simulink model "twr_2017a"  (R2020a)
settings: Solver=FixedStepDiscrete  StartTime=0.0  StopTime=inf  FixedStep=mdl_T_sample  RelTol=1e-3
undefined symbols (not defined in the file or in its folder): ctrl_lqr_addlDyn_A_discrete, ctrl_lqr_addlDyn_B_discrete, ctrl_lqr_addlDyn_C_discrete, ctrl_lqr_addlDyn_D_discrete, ctrl_lqr_addlDyn_k_antiWindup, ctrl_lqr_addlDyn_stateIC, ctrl_lqr_K2, ctrl_motorDriver_v_ff_cmd_v_val, ctrl_motorDriver_v_ff_cmd_v_val_norm_dx_max, ctrl_motorDriver_v_ff_cmd_v_val_norm_dx_min, ctrl_motorDriver_v_output_max, ctrl_motorDriver_v_output_min, ctrl_motorDriver_v_pid_cmd_thetaDot_val, ctrl_motorDriver_v_pid_cmd_thetaDot_val_norm_dx_max, ctrl_motorDriver_v_pid_cmd_thetaDot_val_norm_dx_min, ctrl_motorDriver_v_pid_int_maxVal, ctrl_motorDriver_v_pid_int_minVal, ctrl_motorDriver_v_pid_k_d, ctrl_motorDriver_v_pid_k_i, ctrl_motorDriver_v_pid_k_p, ctrl_motorDriver_v_rts_ss_k_A, ctrl_motorDriver_v_rts_ss_k_B, ctrl_motorDriver_v_rts_ss_k_C, ctrl_motorDriver_v_rts_ss_k_D, ctrl_motorDriver_v_rts_ss_stateIC, ctrl_motorDriver_v_sfr_cmd_p_x_f, ctrl_motorDriver_v_sfr_cmd_p_x_mag, ctrl_motorDriver_v_sfr_cmd_p_y_f, ctrl_motorDriver_v_sfr_cmd_p_y_mag, ctrl_motorDriver_v_sfr_K, ctrl_motorDriver_v_sfr_K_plant, ctrl_motorDriver_v_sfr_K_rts, ctrl_motorDriver_v_T_cmd, ctrl_motorDriver_v_T_init, DiscIntNeverNeededParam, gyro_bias, io_srl_read_rateTransition_initialCondition, k_intmax_uint8, mdl_T_sample, mtr_encoder_filter_z_ss_A, mtr_encoder_filter_z_ss_B, mtr_encoder_filter_z_ss_C, mtr_encoder_filter_z_ss_D, plant, plant_accel_k_digital2analog, plant_body_l_c, plant_body_l_w, plant_gyro_bias_movingAverage_n_pts, plant_gyro_encoder_filter_z_den, plant_gyro_encoder_filter_z_num, plant_gyro_filter_z_den, plant_gyro_filter_z_num, plant_gyro_k_digital2analog, plant_linear_A_continuous, plant_linear_B_continuous, plant_linear_C_continuous, plant_linear_D_continuous, plant_linear_ss_stateIC, plant_linear_ss_t_A, plant_linear_ss_t_B ... (+10)
libraries: svdutilitieslib x135, simulink x57, arduinolib x15, MinSegLibrary_M2V3 x3, dspindex x3, RASPlib x2
(part 5 of 6)

== system twr_2017a/User IO/Writes (To PC)/Plant: Linear Dynamics/Controller: PID/Motor Characterization ==
  note: There is no need to change the datatype paramter
      | listed in the Byte Pack blocks.
      |
      | It will update automatically based on the datatype parameter
      | listed in the Datatype Conversion Block,
      | through the use of the initialization script.
  systemSignalBus : Inport
  Bus Selector : BusSelector  OutputSignals="plant.clock.time [s],io.reads.userInput.controller.output_vMotor.command,plant.encoders.left.angularVelocity  [rad/s],plant.encoders.middle.angularVelocity  [rad/s],controller.motorAngularVelocity.left.voltage.command [V],controller.motorAngularVelocity.middle.voltage.command [V],plant.drivers.left.voltage.command.digital.positive [V],plant.drivers.left.voltage.command.digital.negative [V],plant.drivers.middle.voltage.command.digital.positive [V],plant.drivers.middle.voltage.command.digital.negative [V]"
  Byte Pack - 01 : svdutilitieslib/Byte Pack  datatypes={'single'}  byteAlign=1  blockPlatform=arduinoert
      settings: AttributesFormatString=%<datatypes>  SourceProductName=Simulink Support Package for Arduino Hardware
  Byte Pack - 02 : svdutilitieslib/Byte Pack  datatypes={'single'}  byteAlign=1  blockPlatform=arduinoert
      settings: AttributesFormatString=%<datatypes>  SourceProductName=Simulink Support Package for Arduino Hardware
  Byte Pack - 03 : svdutilitieslib/Byte Pack  datatypes={'single'}  byteAlign=1  blockPlatform=arduinoert
      settings: AttributesFormatString=%<datatypes>  SourceProductName=Simulink Support Package for Arduino Hardware
  Byte Pack - 04 : svdutilitieslib/Byte Pack  datatypes={'single'}  byteAlign=1  blockPlatform=arduinoert
      settings: AttributesFormatString=%<datatypes>  SourceProductName=Simulink Support Package for Arduino Hardware
  Byte Pack - 05 : svdutilitieslib/Byte Pack  datatypes={'single'}  byteAlign=1  blockPlatform=arduinoert
      settings: AttributesFormatString=%<datatypes>  SourceProductName=Simulink Support Package for Arduino Hardware
  Byte Pack - 06 : svdutilitieslib/Byte Pack  datatypes={'single'}  byteAlign=1  blockPlatform=arduinoert
      settings: AttributesFormatString=%<datatypes>  SourceProductName=Simulink Support Package for Arduino Hardware
  Byte Pack - 07 : svdutilitieslib/Byte Pack  datatypes={'single'}  byteAlign=1  blockPlatform=arduinoert
      settings: AttributesFormatString=%<datatypes>  SourceProductName=Simulink Support Package for Arduino Hardware
  Byte Pack - 08 : svdutilitieslib/Byte Pack  datatypes={'single'}  byteAlign=1  blockPlatform=arduinoert
      settings: AttributesFormatString=%<datatypes>  SourceProductName=Simulink Support Package for Arduino Hardware
  Byte Pack - 09 : svdutilitieslib/Byte Pack  datatypes={'uint8'}  byteAlign=1  blockPlatform=arduinoert
      settings: AttributesFormatString=%<datatypes>  SourceProductName=Simulink Support Package for Arduino Hardware
  Byte Pack - 10 : svdutilitieslib/Byte Pack  datatypes={'uint8'}  byteAlign=1  blockPlatform=arduinoert
      settings: AttributesFormatString=%<datatypes>  SourceProductName=Simulink Support Package for Arduino Hardware
  Data Type Conversion - 01 : DataTypeConversion  OutDataTypeStr=single
  Data Type Conversion - 02 : DataTypeConversion  OutDataTypeStr=single
  Data Type Conversion - 03 : DataTypeConversion  OutDataTypeStr=single
  Data Type Conversion - 04 : DataTypeConversion  OutDataTypeStr=single
  Data Type Conversion - 05 : DataTypeConversion  OutDataTypeStr=single
  Data Type Conversion - 06 : DataTypeConversion  OutDataTypeStr=single
  Data Type Conversion - 07 : DataTypeConversion  OutDataTypeStr=uint8
  Data Type Conversion - 08 : DataTypeConversion  OutDataTypeStr=uint8
  Data Type Conversion - 09 : DataTypeConversion  OutDataTypeStr=uint8
  Data Type Conversion - 10 : DataTypeConversion  OutDataTypeStr=uint8
  Mux : Mux  Inputs=10
  Rate Transition : RateTransition  InitialCondition=io_srl_read_rateTransition_initialCondition  OutPortSampleTimeMultiple=io_read_rateTransition_decimation  OutPortSampleTime=io_srl_read_rateTransition_T_sample
      settings: AttributesFormatString=|
      | Output sample time: %<OutPortSampleTime>
      | Initial condition: %<X0>
  Serial Transmit : arduinolib/Serial Transmit  portNumber=0  sendmode=write  sendformat=Decimal  floatprecision=2  blockPlatform=arduino
  wires:
  Bus Selector/1 -> Data Type Conversion - 01/1  "<time [s]>"
  Rate Transition/1 -> Serial Transmit/1
  Bus Selector/4 -> Data Type Conversion - 04/1  "<angularVelocity  [rad/s]>"
  Bus Selector/3 -> Data Type Conversion - 03/1  "<angularVelocity  [rad/s]>"
  Data Type Conversion - 10/1 -> Byte Pack - 10/1
  Data Type Conversion - 09/1 -> Byte Pack - 09/1
  Data Type Conversion - 08/1 -> Byte Pack - 08/1
  Data Type Conversion - 07/1 -> Byte Pack - 07/1
  Data Type Conversion - 06/1 -> Byte Pack - 06/1
  Data Type Conversion - 05/1 -> Byte Pack - 05/1
  Data Type Conversion - 04/1 -> Byte Pack - 04/1
  Data Type Conversion - 03/1 -> Byte Pack - 03/1
  Data Type Conversion - 02/1 -> Byte Pack - 02/1
  Data Type Conversion - 01/1 -> Byte Pack - 01/1
  Byte Pack - 10/1 -> Mux/10
  Byte Pack - 09/1 -> Mux/9
  Bus Selector/2 -> Data Type Conversion - 02/1  "<command>"
  systemSignalBus/1 -> Bus Selector/1
  Byte Pack - 02/1 -> Mux/2
  Byte Pack - 08/1 -> Mux/8
  Byte Pack - 05/1 -> Mux/5
  Byte Pack - 06/1 -> Mux/6
  Byte Pack - 01/1 -> Mux/1
  Mux/1 -> Rate Transition/1
  Byte Pack - 07/1 -> Mux/7
  Byte Pack - 03/1 -> Mux/3
  Byte Pack - 04/1 -> Mux/4
  Bus Selector/5 -> Data Type Conversion - 05/1  "<command [V]>"
  Bus Selector/6 -> Data Type Conversion - 06/1  "<command [V]>"
  Bus Selector/7 -> Data Type Conversion - 07/1  "<positive [V]>"
  Bus Selector/8 -> Data Type Conversion - 08/1  "<negative [V]>"
  Bus Selector/9 -> Data Type Conversion - 09/1  "<positive [V]>"
  Bus Selector/10 -> Data Type Conversion - 10/1  "<negative [V]>"

== system twr_2017a/User IO/Writes (To PC)/Plant: Linear Dynamics/Controller: PID/Standard ==
  systemSignalBus : Inport
  Bus Creator : BusCreator  Inputs=4
  Bus Selector : BusSelector  OutputSignals=userIO.read.controller.command.theta_body_average [rad],plant.position.theta.global.average.position [rad],controller.error.motorDriver.error.theta_body_average [rad]
  Bus Selector1 : BusSelector  OutputSignals=userIO.read.controller.command.phi_y [rad],plant.position.phi.y (yaw).position [rad],controller.error.motorDriver.error.phi_y [rad]
  Bus Selector2 : BusSelector  OutputSignals=plant.position.phi.x (pitch).position [rad]
  Bus Selector3 : BusSelector  OutputSignals="controller.output.motorDriver.left.voltage.command  [V],controller.output.motorDriver.middle.voltage.command [V]"
  Bus Selector4 : BusSelector  OutputSignals=plant.position.p.wheel.center.x.position [m],plant.position.p.wheel.center.y.position [m]
  Bus Selector5 : BusSelector  OutputSignals=plant.position.p.wheel.center.x.position [m],plant.position.p.wheel.center.y.position [m]
  Bus Selector6 : BusSelector  OutputSignals=userIO.read.controller.command.theta_body_average [rad],userIO.read.controller.command.phi_y [rad]
  Bus Selector7 : BusSelector  OutputSignals=x.position [m],y.position [m]
  Bus Selector8 : BusSelector  OutputSignals=plant.position.p.wheel.center.x.position [m],plant.position.p.wheel.center.y.position [m]
  Discrete Derivative : simulink/Discrete/Discrete Derivative  gainval=1.0  ICPrevScaledInput=0.0  OutMin=[]  OutMax=[]  OutDataType=fixdt(1, 16)  OutScaling=2^-10  DoSatur=off
  Pass Through : Subsystem
  To Workspace : ToWorkspace  VariableName=xy  SaveFormat=Timeseries  SampleTime=-1
  Wheel : Subsystem
  XY Graph : simulink/Sinks/XY Graph  xmin=-1  xmax=+1  ymin=-1  ymax=+1  st=-1
  pitch : Scope
  theta : Scope  NumInputPorts=3
  v.lm : Scope  NumInputPorts=2
  xy : Scope  NumInputPorts=2
  yaw : Scope  NumInputPorts=3
  wires:
  Bus Selector/1 -> theta/1  "<theta_body_average [rad]>"
  Bus Selector/2 -> theta/2  "<position [rad]>"
  Bus Selector/3 -> theta/3  "<theta_body_average [rad]>"
  Bus Selector1/1 -> yaw/1  "<phi_y [rad]>"
  Bus Selector1/2 -> yaw/2  "<position [rad]>"
  Bus Selector1/3 -> yaw/3  "<phi_y [rad]>"
  Bus Selector2/1 -> pitch/1  "<position [rad]>"
  Bus Selector3/1 -> v.lm/1  "<command  [V]>"
  Bus Selector3/2 -> v.lm/2  "<command [V]>"
  Bus Selector5/1 -> xy/1  "<position [m]>"
  Bus Selector5/2 -> xy/2  "<position [m]>"
  Bus Selector4/2 -> XY Graph/2  "<position [m]>"
  Bus Selector4/1 -> XY Graph/1  "<position [m]>"
  Bus Selector6/1 -> Discrete Derivative/1  "<theta_body_average [rad]>"
  Bus Selector6/2 -> Wheel/2(body.angularPosition.y (yaw))  "<phi_y [rad]>"
  Wheel/3(center) -> Bus Selector7/1
  Discrete Derivative/1 -> Wheel/1(wheel.angularVelocity.global)
  systemSignalBus/1 -> Bus Selector5/1, Bus Selector4/1, Bus Selector6/1, Bus Selector8/1, Bus Selector3/1, Bus Selector2/1, Bus Selector1/1, Bus Selector/1
  Pass Through/4(Out4) -> Bus Creator/4  "act.y"
  Pass Through/3(Out3) -> Bus Creator/3  "act.x"
  Pass Through/2(Out2) -> Bus Creator/2  "ref.y"
  Pass Through/1(Out1) -> Bus Creator/1  "ref.x"
  Bus Creator/1 -> To Workspace/1
  Bus Selector7/1 -> Pass Through/1(In1)  "<position [m]>"
  Bus Selector7/2 -> Pass Through/2(In2)  "<position [m]>"
  Bus Selector8/1 -> Pass Through/3(In3)  "<position [m]>"
  Bus Selector8/2 -> Pass Through/4(In4)  "<position [m]>"

== system twr_2017a/User IO/Writes (To PC)/Plant: Linear Dynamics/Controller: SFR/Error ==
  x.command.in : Inport
  y.command.in : Inport  Port=2
  x.actual.in : Inport  Port=3
  y.actual.in : Inport  Port=4
  Add : Sum  Inputs=+-
  Add1 : Sum  Inputs=+-
  x.command : Outport
  x.actual : Outport  Port=2
  x.error : Outport  Port=3
  y.command : Outport  Port=4
  y.actual : Outport  Port=5
  y.error : Outport  Port=6
  wires:
  x.command.in/1 -> [x_cmd]
  x.actual.in/1 -> [x_act]
  y.command.in/1 -> [y_cmd]
  y.actual.in/1 -> [y_act]
  [x_cmd] -> x.command/1
  [x_act] -> x.actual/1
  [y_cmd] -> y.command/1
  [y_act] -> y.actual/1
  Add/1 -> y.error/1
  [y_cmd] -> Add/1
  [y_act] -> Add/2
  [x_act] -> Add1/2
  [x_cmd] -> Add1/1
  Add1/1 -> x.error/1

== system twr_2017a/User IO/Writes (To PC)/Plant: Nonlinear Dynamics/Controller: FF/Standard ==
  note: There is no need to change the datatype paramter
      | listed in the Byte Pack blocks.
      |
      | It will update automatically based on the datatype parameter
      | listed in the Datatype Conversion Block,
      | through the use of the initialization script.
  systemSignalBus : Inport
  Bus Selector : BusSelector  OutputSignals="plant.clock.time [s],io.reads.userInput.command,plant.encoders.left.angularVelocity  [rad/s],plant.encoders.middle.angularVelocity  [rad/s],controller.motorAngularVelocity.left.voltage.command [V],controller.motorAngularVelocity.middle.voltage.command [V],plant.drivers.left.voltage.command.digital.positive [V],plant.drivers.left.voltage.command.digital.negative [V],plant.drivers.middle.voltage.command.digital.positive [V],plant.drivers.middle.voltage.command.digital.negative [V],plant.gyroscope.x.w [rad/s],plant.gyroscope.x.theta [rad],plant.gyroscope.y.w [rad/s],plant.gyroscope.y.theta [rad],plant.gyroscope.z.w [rad/s],plant.gyroscope.z.theta [rad]"
  Byte Pack - 01 : svdutilitieslib/Byte Pack  datatypes={'single'}  byteAlign=1  blockPlatform=arduinoert
      settings: AttributesFormatString=%<datatypes>  SourceProductName=Simulink Support Package for Arduino Hardware
  Byte Pack - 02 : svdutilitieslib/Byte Pack  datatypes={'single'}  byteAlign=1  blockPlatform=arduinoert
      settings: AttributesFormatString=%<datatypes>  SourceProductName=Simulink Support Package for Arduino Hardware
  Byte Pack - 03 : svdutilitieslib/Byte Pack  datatypes={'single'}  byteAlign=1  blockPlatform=arduinoert
      settings: AttributesFormatString=%<datatypes>  SourceProductName=Simulink Support Package for Arduino Hardware
  Byte Pack - 04 : svdutilitieslib/Byte Pack  datatypes={'single'}  byteAlign=1  blockPlatform=arduinoert
      settings: AttributesFormatString=%<datatypes>  SourceProductName=Simulink Support Package for Arduino Hardware
  Byte Pack - 05 : svdutilitieslib/Byte Pack  datatypes={'single'}  byteAlign=1  blockPlatform=arduinoert
      settings: AttributesFormatString=%<datatypes>  SourceProductName=Simulink Support Package for Arduino Hardware
  Byte Pack - 06 : svdutilitieslib/Byte Pack  datatypes={'single'}  byteAlign=1  blockPlatform=arduinoert
      settings: AttributesFormatString=%<datatypes>  SourceProductName=Simulink Support Package for Arduino Hardware
  Byte Pack - 07 : svdutilitieslib/Byte Pack  datatypes={'single'}  byteAlign=1  blockPlatform=arduinoert
      settings: AttributesFormatString=%<datatypes>  SourceProductName=Simulink Support Package for Arduino Hardware
  Byte Pack - 08 : svdutilitieslib/Byte Pack  datatypes={'single'}  byteAlign=1  blockPlatform=arduinoert
      settings: AttributesFormatString=%<datatypes>  SourceProductName=Simulink Support Package for Arduino Hardware
  Byte Pack - 09 : svdutilitieslib/Byte Pack  datatypes={'uint8'}  byteAlign=1  blockPlatform=arduinoert
      settings: AttributesFormatString=%<datatypes>  SourceProductName=Simulink Support Package for Arduino Hardware
  Byte Pack - 10 : svdutilitieslib/Byte Pack  datatypes={'uint8'}  byteAlign=1  blockPlatform=arduinoert
      settings: AttributesFormatString=%<datatypes>  SourceProductName=Simulink Support Package for Arduino Hardware
  Byte Pack - 11 : svdutilitieslib/Byte Pack  datatypes={'uint8'}  byteAlign=1  blockPlatform=arduinoert
      settings: AttributesFormatString=%<datatypes>  SourceProductName=Simulink Support Package for Arduino Hardware
  Byte Pack - 12 : svdutilitieslib/Byte Pack  datatypes={'uint8'}  byteAlign=1  blockPlatform=arduinoert
      settings: AttributesFormatString=%<datatypes>  SourceProductName=Simulink Support Package for Arduino Hardware
  Byte Pack - 13 : svdutilitieslib/Byte Pack  datatypes={'single'}  byteAlign=1  blockPlatform=arduinoert
      settings: AttributesFormatString=%<datatypes>  SourceProductName=Simulink Support Package for Arduino Hardware
  Byte Pack - 14 : svdutilitieslib/Byte Pack  datatypes={'single'}  byteAlign=1  blockPlatform=arduinoert
      settings: AttributesFormatString=%<datatypes>  SourceProductName=Simulink Support Package for Arduino Hardware
  Data Type Conversion - 01 : DataTypeConversion  OutDataTypeStr=single
  Data Type Conversion - 02 : DataTypeConversion  OutDataTypeStr=single
  Data Type Conversion - 03 : DataTypeConversion  OutDataTypeStr=single
  Data Type Conversion - 04 : DataTypeConversion  OutDataTypeStr=single
  Data Type Conversion - 05 : DataTypeConversion  OutDataTypeStr=single
  Data Type Conversion - 06 : DataTypeConversion  OutDataTypeStr=single
  Data Type Conversion - 07 : DataTypeConversion  OutDataTypeStr=single
  Data Type Conversion - 08 : DataTypeConversion  OutDataTypeStr=single
  Data Type Conversion - 09 : DataTypeConversion  OutDataTypeStr=uint8
  Data Type Conversion - 10 : DataTypeConversion  OutDataTypeStr=uint8
  Data Type Conversion - 11 : DataTypeConversion  OutDataTypeStr=uint8
  Data Type Conversion - 12 : DataTypeConversion  OutDataTypeStr=uint8
  Data Type Conversion - 13 : DataTypeConversion  OutDataTypeStr=single
  Data Type Conversion - 14 : DataTypeConversion  OutDataTypeStr=single
  Mux : Mux  Inputs=14
  Rate Transition : RateTransition  InitialCondition=io_srl_read_rateTransition_initialCondition  OutPortSampleTimeMultiple=io_read_rateTransition_decimation  OutPortSampleTime=io_srl_read_rateTransition_T_sample
      settings: AttributesFormatString=|
      | Output sample time: %<OutPortSampleTime>
      | Initial condition: %<X0>
  Serial Transmit : arduinolib/Serial Transmit  portNumber=0  sendmode=write  sendformat=Decimal  floatprecision=2  blockPlatform=arduino
  wires:
  Bus Selector/1 -> Data Type Conversion - 01/1  "<time [s]>"
  Byte Pack - 14/1 -> Mux/14
  Bus Selector/12 -> Data Type Conversion - 14/1  "<theta [rad]>"
  Data Type Conversion - 14/1 -> Byte Pack - 14/1
  Bus Selector/11 -> Data Type Conversion - 13/1  "<w [rad/s]>"
  Data Type Conversion - 13/1 -> Byte Pack - 13/1
  Byte Pack - 13/1 -> Mux/13
  Rate Transition/1 -> Serial Transmit/1
  Bus Selector/6 -> Data Type Conversion - 08/1  "<command [V]>"
  Bus Selector/5 -> Data Type Conversion - 07/1  "<command [V]>"
  ? -> Data Type Conversion - 06/1  "<error [rad/s]>"
  ? -> Data Type Conversion - 05/1  "<error [rad/s]>"
  Bus Selector/4 -> Data Type Conversion - 04/1  "<angularVelocity  [rad/s]>"
  Bus Selector/3 -> Data Type Conversion - 03/1  "<angularVelocity  [rad/s]>"
  Byte Pack - 12/1 -> Mux/12
  Byte Pack - 11/1 -> Mux/11
  Bus Selector/9 -> Data Type Conversion - 11/1  "<positive [V]>"
  Bus Selector/10 -> Data Type Conversion - 12/1  "<negative [V]>"
  Data Type Conversion - 11/1 -> Byte Pack - 11/1
  Data Type Conversion - 12/1 -> Byte Pack - 12/1
  Data Type Conversion - 10/1 -> Byte Pack - 10/1
  Data Type Conversion - 09/1 -> Byte Pack - 09/1
  Data Type Conversion - 08/1 -> Byte Pack - 08/1
  Data Type Conversion - 07/1 -> Byte Pack - 07/1
  Data Type Conversion - 06/1 -> Byte Pack - 06/1
  Data Type Conversion - 05/1 -> Byte Pack - 05/1
  Data Type Conversion - 04/1 -> Byte Pack - 04/1
  Data Type Conversion - 03/1 -> Byte Pack - 03/1
  Data Type Conversion - 02/1 -> Byte Pack - 02/1
  Data Type Conversion - 01/1 -> Byte Pack - 01/1
  Byte Pack - 10/1 -> Mux/10
  Byte Pack - 09/1 -> Mux/9
  Bus Selector/8 -> Data Type Conversion - 10/1  "<negative [V]>"
  Bus Selector/7 -> Data Type Conversion - 09/1  "<positive [V]>"
  Bus Selector/2 -> Data Type Conversion - 02/1  "<command>"
  systemSignalBus/1 -> Bus Selector/1
  Byte Pack - 02/1 -> Mux/2
  Byte Pack - 08/1 -> Mux/8
  Byte Pack - 05/1 -> Mux/5
  Byte Pack - 06/1 -> Mux/6
  Byte Pack - 01/1 -> Mux/1
  Mux/1 -> Rate Transition/1
  Byte Pack - 07/1 -> Mux/7
  Byte Pack - 03/1 -> Mux/3
  Byte Pack - 04/1 -> Mux/4

== system twr_2017a/User IO/Writes (To PC)/Plant: Nonlinear Dynamics/Controller: PID/Standard ==
  note: There is no need to change the datatype paramter
      | listed in the Byte Pack blocks.
      |
      | It will update automatically based on the datatype parameter
      | listed in the Datatype Conversion Block,
      | through the use of the initialization script.
  systemSignalBus : Inport
  Bus Selector : BusSelector  OutputSignals="plant.clock.time [s],io.reads.userInput.command,plant.encoders.left.angularVelocity  [rad/s],plant.encoders.middle.angularVelocity  [rad/s],controller.motorAngularVelocity.left.voltage.command [V],controller.motorAngularVelocity.middle.voltage.command [V],plant.drivers.left.voltage.command.digital.positive [V],plant.drivers.left.voltage.command.digital.negative [V],plant.drivers.middle.voltage.command.digital.positive [V],plant.drivers.middle.voltage.command.digital.negative [V],plant.gyroscope.x.w [rad/s],plant.gyroscope.x.theta [rad],plant.gyroscope.y.w [rad/s],plant.gyroscope.y.theta [rad],plant.gyroscope.z.w [rad/s],plant.gyroscope.z.theta [rad]"
  Byte Pack - 01 : svdutilitieslib/Byte Pack  datatypes={'single'}  byteAlign=1  blockPlatform=arduinoert
      settings: AttributesFormatString=%<datatypes>  SourceProductName=Simulink Support Package for Arduino Hardware
  Byte Pack - 02 : svdutilitieslib/Byte Pack  datatypes={'single'}  byteAlign=1  blockPlatform=arduinoert
      settings: AttributesFormatString=%<datatypes>  SourceProductName=Simulink Support Package for Arduino Hardware
  Byte Pack - 03 : svdutilitieslib/Byte Pack  datatypes={'single'}  byteAlign=1  blockPlatform=arduinoert
      settings: AttributesFormatString=%<datatypes>  SourceProductName=Simulink Support Package for Arduino Hardware
  Byte Pack - 04 : svdutilitieslib/Byte Pack  datatypes={'single'}  byteAlign=1  blockPlatform=arduinoert
      settings: AttributesFormatString=%<datatypes>  SourceProductName=Simulink Support Package for Arduino Hardware
  Byte Pack - 05 : svdutilitieslib/Byte Pack  datatypes={'single'}  byteAlign=1  blockPlatform=arduinoert
      settings: AttributesFormatString=%<datatypes>  SourceProductName=Simulink Support Package for Arduino Hardware
  Byte Pack - 06 : svdutilitieslib/Byte Pack  datatypes={'single'}  byteAlign=1  blockPlatform=arduinoert
      settings: AttributesFormatString=%<datatypes>  SourceProductName=Simulink Support Package for Arduino Hardware
  Byte Pack - 07 : svdutilitieslib/Byte Pack  datatypes={'single'}  byteAlign=1  blockPlatform=arduinoert
      settings: AttributesFormatString=%<datatypes>  SourceProductName=Simulink Support Package for Arduino Hardware
  Byte Pack - 08 : svdutilitieslib/Byte Pack  datatypes={'single'}  byteAlign=1  blockPlatform=arduinoert
      settings: AttributesFormatString=%<datatypes>  SourceProductName=Simulink Support Package for Arduino Hardware
  Byte Pack - 09 : svdutilitieslib/Byte Pack  datatypes={'uint8'}  byteAlign=1  blockPlatform=arduinoert
      settings: AttributesFormatString=%<datatypes>  SourceProductName=Simulink Support Package for Arduino Hardware
  Byte Pack - 10 : svdutilitieslib/Byte Pack  datatypes={'uint8'}  byteAlign=1  blockPlatform=arduinoert
      settings: AttributesFormatString=%<datatypes>  SourceProductName=Simulink Support Package for Arduino Hardware
  Byte Pack - 11 : svdutilitieslib/Byte Pack  datatypes={'uint8'}  byteAlign=1  blockPlatform=arduinoert
      settings: AttributesFormatString=%<datatypes>  SourceProductName=Simulink Support Package for Arduino Hardware
  Byte Pack - 12 : svdutilitieslib/Byte Pack  datatypes={'uint8'}  byteAlign=1  blockPlatform=arduinoert
      settings: AttributesFormatString=%<datatypes>  SourceProductName=Simulink Support Package for Arduino Hardware
  Byte Pack - 13 : svdutilitieslib/Byte Pack  datatypes={'single'}  byteAlign=1  blockPlatform=arduinoert
      settings: AttributesFormatString=%<datatypes>  SourceProductName=Simulink Support Package for Arduino Hardware
  Byte Pack - 14 : svdutilitieslib/Byte Pack  datatypes={'single'}  byteAlign=1  blockPlatform=arduinoert
      settings: AttributesFormatString=%<datatypes>  SourceProductName=Simulink Support Package for Arduino Hardware
  Data Type Conversion - 01 : DataTypeConversion  OutDataTypeStr=single
  Data Type Conversion - 02 : DataTypeConversion  OutDataTypeStr=single
  Data Type Conversion - 03 : DataTypeConversion  OutDataTypeStr=single
  Data Type Conversion - 04 : DataTypeConversion  OutDataTypeStr=single
  Data Type Conversion - 05 : DataTypeConversion  OutDataTypeStr=single
  Data Type Conversion - 06 : DataTypeConversion  OutDataTypeStr=single
  Data Type Conversion - 07 : DataTypeConversion  OutDataTypeStr=single
  Data Type Conversion - 08 : DataTypeConversion  OutDataTypeStr=single
  Data Type Conversion - 09 : DataTypeConversion  OutDataTypeStr=uint8
  Data Type Conversion - 10 : DataTypeConversion  OutDataTypeStr=uint8
  Data Type Conversion - 11 : DataTypeConversion  OutDataTypeStr=uint8
  Data Type Conversion - 12 : DataTypeConversion  OutDataTypeStr=uint8
  Data Type Conversion - 13 : DataTypeConversion  OutDataTypeStr=single
  Data Type Conversion - 14 : DataTypeConversion  OutDataTypeStr=single
  Mux : Mux  Inputs=14
  Rate Transition : RateTransition  InitialCondition=io_srl_read_rateTransition_initialCondition  OutPortSampleTimeMultiple=io_read_rateTransition_decimation  OutPortSampleTime=io_srl_read_rateTransition_T_sample
      settings: AttributesFormatString=|
      | Output sample time: %<OutPortSampleTime>
      | Initial condition: %<X0>
  Serial Transmit : arduinolib/Serial Transmit  portNumber=0  sendmode=write  sendformat=Decimal  floatprecision=2  blockPlatform=arduino
  wires:
  Byte Pack - 04/1 -> Mux/4
  Byte Pack - 03/1 -> Mux/3
  Byte Pack - 07/1 -> Mux/7
  Mux/1 -> Rate Transition/1
  Byte Pack - 01/1 -> Mux/1
  Byte Pack - 06/1 -> Mux/6
  Byte Pack - 05/1 -> Mux/5
  Byte Pack - 08/1 -> Mux/8
  Byte Pack - 02/1 -> Mux/2
  systemSignalBus/1 -> Bus Selector/1
  Bus Selector/2 -> Data Type Conversion - 02/1  "<command>"
  Bus Selector/7 -> Data Type Conversion - 09/1  "<positive [V]>"
  Bus Selector/8 -> Data Type Conversion - 10/1  "<negative [V]>"
  Byte Pack - 09/1 -> Mux/9
  Byte Pack - 10/1 -> Mux/10
  Data Type Conversion - 01/1 -> Byte Pack - 01/1
  Data Type Conversion - 02/1 -> Byte Pack - 02/1
  Data Type Conversion - 03/1 -> Byte Pack - 03/1
  Data Type Conversion - 04/1 -> Byte Pack - 04/1
  Data Type Conversion - 05/1 -> Byte Pack - 05/1
  Data Type Conversion - 06/1 -> Byte Pack - 06/1
  Data Type Conversion - 07/1 -> Byte Pack - 07/1
  Data Type Conversion - 08/1 -> Byte Pack - 08/1
  Data Type Conversion - 09/1 -> Byte Pack - 09/1
  Data Type Conversion - 10/1 -> Byte Pack - 10/1
  Data Type Conversion - 12/1 -> Byte Pack - 12/1
  Data Type Conversion - 11/1 -> Byte Pack - 11/1
  Bus Selector/10 -> Data Type Conversion - 12/1  "<negative [V]>"
  Bus Selector/9 -> Data Type Conversion - 11/1  "<positive [V]>"
  Byte Pack - 11/1 -> Mux/11
  Byte Pack - 12/1 -> Mux/12
  Bus Selector/3 -> Data Type Conversion - 03/1  "<angularVelocity  [rad/s]>"
  Bus Selector/4 -> Data Type Conversion - 04/1  "<angularVelocity  [rad/s]>"
  ? -> Data Type Conversion - 05/1  "<error [rad/s]>"
  ? -> Data Type Conversion - 06/1  "<error [rad/s]>"
  Bus Selector/5 -> Data Type Conversion - 07/1  "<command [V]>"
  Bus Selector/6 -> Data Type Conversion - 08/1  "<command [V]>"
  Rate Transition/1 -> Serial Transmit/1
  Byte Pack - 13/1 -> Mux/13
  Data Type Conversion - 13/1 -> Byte Pack - 13/1
  Bus Selector/11 -> Data Type Conversion - 13/1  "<w [rad/s]>"
  Data Type Conversion - 14/1 -> Byte Pack - 14/1
  Bus Selector/12 -> Data Type Conversion - 14/1  "<theta [rad]>"
  Byte Pack - 14/1 -> Mux/14
  Bus Selector/1 -> Data Type Conversion - 01/1  "<time [s]>"

== system twr_2017a/Controller [v.motorDriver]/Archive/Additional Dynamics: Reference Tracking/Delay/x1/Saturation flag ==
  u[k+1] : Inport
  u.max : Inport  Port=2
  u.min : Inport  Port=3
  Add : Sum
  Data Type Conversion : DataTypeConversion  OutDataTypeStr=uint8
  Data Type Conversion1 : DataTypeConversion  OutDataTypeStr=uint8
  Gain : Gain  Gain=uint8(1)  OutDataTypeStr=uint8
      settings: AttributesFormatString=%<Gain>
  Gain1 : Gain  Gain=uint8(2)  OutDataTypeStr=uint8
      settings: AttributesFormatString=%<Gain>
  Relational Operator : RelationalOperator  OutDataTypeStr=boolean  RndMeth=Nearest
  Relational Operator1 : RelationalOperator  Operator=<=  OutDataTypeStr=boolean  RndMeth=Nearest
  x.saturating : Outport
  wires:
  u[k+1]/1 -> [u_kp1]
  [u_kp1] -> Relational Operator/1
  u.max/1 -> Relational Operator/2
  [u_kp1] -> Relational Operator1/1
  u.min/1 -> Relational Operator1/2
  Add/1 -> x.saturating/1  "x.saturating"
  Relational Operator1/1 -> Data Type Conversion1/1  "x.lowerSaturating"
  Relational Operator/1 -> Data Type Conversion/1  "x.upperSaturating"
  Data Type Conversion/1 -> Gain/1
  Data Type Conversion1/1 -> Gain1/1
  Gain/1 -> Add/1
  Gain1/1 -> Add/2

== system twr_2017a/Controller [v.motorDriver]/Archive/Additional Dynamics: Reference Tracking/Delay/x1/anti-windup ==
  u[k+1].preSat.in : Inport
  u[k+1].postSat.in : Inport  Port=2
  Add : Sum  Inputs=-+
  Add1 : Sum
  Gain : Gain  Gain=k_antiWindup
      settings: AttributesFormatString=%<Gain>
  u[k+1].postSat.out : Outport
  wires:
  Add1/1 -> u[k+1].postSat.out/1
  Add/1 -> Gain/1
  u[k+1].preSat.in/1 -> Add/1, Add1/1
  u[k+1].postSat.in/1 -> Add/2
  Gain/1 -> Add1/2

== system twr_2017a/Controller [v.motorDriver]/Archive/Additional Dynamics: Reference Tracking/Delay/x2/Saturation flag ==
  u[k+1] : Inport
  u.max : Inport  Port=2
  u.min : Inport  Port=3
  Add : Sum
  Data Type Conversion : DataTypeConversion  OutDataTypeStr=uint8
  Data Type Conversion1 : DataTypeConversion  OutDataTypeStr=uint8
  Gain : Gain  Gain=uint8(1)  OutDataTypeStr=uint8
      settings: AttributesFormatString=%<Gain>
  Gain1 : Gain  Gain=uint8(2)  OutDataTypeStr=uint8
      settings: AttributesFormatString=%<Gain>
  Relational Operator : RelationalOperator  OutDataTypeStr=boolean  RndMeth=Nearest
  Relational Operator1 : RelationalOperator  Operator=<=  OutDataTypeStr=boolean  RndMeth=Nearest
  x.saturating : Outport
  wires:
  Gain1/1 -> Add/2
  Gain/1 -> Add/1
  Data Type Conversion1/1 -> Gain1/1
  Data Type Conversion/1 -> Gain/1
  Relational Operator/1 -> Data Type Conversion/1  "x.upperSaturating"
  Relational Operator1/1 -> Data Type Conversion1/1  "x.lowerSaturating"
  Add/1 -> x.saturating/1  "x.saturating"
  u.min/1 -> Relational Operator1/2
  [u_kp1] -> Relational Operator1/1
  u.max/1 -> Relational Operator/2
  [u_kp1] -> Relational Operator/1
  u[k+1]/1 -> [u_kp1]

== system twr_2017a/Controller [v.motorDriver]/Archive/Additional Dynamics: Reference Tracking/Delay/x2/anti-windup ==
  u[k+1].preSat.in : Inport
  u[k+1].postSat.in : Inport  Port=2
  Add : Sum  Inputs=-+
  Add1 : Sum
  Gain : Gain  Gain=k_antiWindup
      settings: AttributesFormatString=%<Gain>
  u[k+1].postSat.out : Outport
  wires:
  Gain/1 -> Add1/2
  u[k+1].postSat.in/1 -> Add/2
  u[k+1].preSat.in/1 -> Add1/1, Add/1
  Add/1 -> Gain/1
  Add1/1 -> u[k+1].postSat.out/1

== system twr_2017a/Controller [v.motorDriver]/Archive/Continuous State-Space/Integrator/x1/Saturation flag ==
  u.dot : Inport
  u.max : Inport  Port=2
  u.noSat : Inport  Port=3
  u.min : Inport  Port=4
  Compare To Zero : simulink/Logic and Bit Operations/Compare To Zero  relop=<  OutDataTypeStr=uint8  ZeroCross=off
  Compare To Zero1 : simulink/Logic and Bit Operations/Compare To Zero  relop=>  OutDataTypeStr=uint8  ZeroCross=off
  Logical Operator : Logic  Operator=OR  AllPortsSameDT=off  OutDataTypeStr=boolean
  Logical Operator1 : Logic  Operator=OR  AllPortsSameDT=off  OutDataTypeStr=boolean
  Logical Operator2 : Logic  AllPortsSameDT=off  OutDataTypeStr=boolean
  Logical Operator3 : Logic  Operator=NOT  AllPortsSameDT=off  OutDataTypeStr=boolean
  Relational Operator : RelationalOperator  Operator=<=  OutDataTypeStr=boolean  RndMeth=Nearest
  Relational Operator1 : RelationalOperator  OutDataTypeStr=boolean  RndMeth=Nearest
  x.saturating : Outport
  wires:
  Logical Operator3/1 -> x.saturating/1  "x.saturating"
  [u_min] -> Relational Operator1/2
  [u_noSat] -> Relational Operator1/1
  [u_max] -> Relational Operator/2
  [u_noSat] -> Relational Operator/1
  [u_dot] -> Compare To Zero/1
  [u_dot] -> Compare To Zero1/1
  u.noSat/1 -> [u_noSat]
  Logical Operator2/1 -> Logical Operator3/1  "x.notSaturating"
  Logical Operator/1 -> Logical Operator2/1
  Logical Operator1/1 -> Logical Operator2/2
  Relational Operator1/1 -> Logical Operator1/1
  Compare To Zero1/1 -> Logical Operator1/2
  Compare To Zero/1 -> Logical Operator/2
  Relational Operator/1 -> Logical Operator/1
  u.max/1 -> [u_max]
  u.dot/1 -> [u_dot]
  u.min/1 -> [u_min]

== system twr_2017a/Controller [v.motorDriver]/Archive/Continuous State-Space/Integrator/x2/Saturation flag ==
  u.dot : Inport
  u.max : Inport  Port=2
  u.noSat : Inport  Port=3
  u.min : Inport  Port=4
  Compare To Zero : simulink/Logic and Bit Operations/Compare To Zero  relop=<  OutDataTypeStr=uint8  ZeroCross=off
  Compare To Zero1 : simulink/Logic and Bit Operations/Compare To Zero  relop=>  OutDataTypeStr=uint8  ZeroCross=off
  Logical Operator : Logic  Operator=OR  AllPortsSameDT=off  OutDataTypeStr=boolean
  Logical Operator1 : Logic  Operator=OR  AllPortsSameDT=off  OutDataTypeStr=boolean
  Logical Operator2 : Logic  AllPortsSameDT=off  OutDataTypeStr=boolean
  Logical Operator3 : Logic  Operator=NOT  AllPortsSameDT=off  OutDataTypeStr=boolean
  Relational Operator : RelationalOperator  Operator=<=  OutDataTypeStr=boolean  RndMeth=Nearest
  Relational Operator1 : RelationalOperator  OutDataTypeStr=boolean  RndMeth=Nearest
  x.saturating : Outport
  wires:
  u.min/1 -> [u_min]
  u.dot/1 -> [u_dot]
  u.max/1 -> [u_max]
  Relational Operator/1 -> Logical Operator/1
  Compare To Zero/1 -> Logical Operator/2
  Compare To Zero1/1 -> Logical Operator1/2
  Relational Operator1/1 -> Logical Operator1/1
  Logical Operator1/1 -> Logical Operator2/2
  Logical Operator/1 -> Logical Operator2/1
  Logical Operator2/1 -> Logical Operator3/1  "x.notSaturating"
  u.noSat/1 -> [u_noSat]
  [u_dot] -> Compare To Zero1/1
  [u_dot] -> Compare To Zero/1
  [u_noSat] -> Relational Operator/1
  [u_max] -> Relational Operator/2
  [u_noSat] -> Relational Operator1/1
  [u_min] -> Relational Operator1/2
  Logical Operator3/1 -> x.saturating/1  "x.saturating"

== system twr_2017a/Plant/Hardware/Arduino Pin IO/Digital Outputs (Writes to Pins)/Motor/Left-Connected ==
  motor.left.voltage.command.digital.positive : Inport
  motor.left.voltage.command.digital.negative : Inport  Port=2
  Digital Output (PWM): Pin 6 Motor Driver - Voltage Command (Positive) : arduinolib/PWM  pinNumber=6  blockPlatform=arduino
  Digital Output (PWM): Pin 8 Motor Driver - Voltage Command (Negative) : arduinolib/PWM  pinNumber=8  blockPlatform=arduino
  wires:
  motor.left.voltage.command.digital.negative/1 -> Digital Output (PWM): Pin 8 Motor Driver - Voltage Command (Negative)/1
  motor.left.voltage.command.digital.positive/1 -> Digital Output (PWM): Pin 6 Motor Driver - Voltage Command (Positive)/1

== system twr_2017a/Plant/Hardware/Arduino Pin IO/Digital Outputs (Writes to Pins)/Motor/Right-Connected ==
  motor.middle.voltage.command.digital.positive : Inport
  motor.middle.voltage.command.digital.negative : Inport  Port=2
  Digital Output (PWM): Pin 2 Motor Driver - Voltage Command (Positive) : arduinolib/PWM  pinNumber=2  blockPlatform=arduino
  Digital Output (PWM): Pin 5 Motor Driver - Voltage Command (Negative) : arduinolib/PWM  pinNumber=5  blockPlatform=arduino
  wires:
  motor.middle.voltage.command.digital.positive/1 -> Digital Output (PWM): Pin 2 Motor Driver - Voltage Command (Positive)/1
  motor.middle.voltage.command.digital.negative/1 -> Digital Output (PWM): Pin 5 Motor Driver - Voltage Command (Negative)/1

== system twr_2017a/Plant/Hardware/Calculations/Body Angular Position (phi)/X (Pitch)/Accelerometer ==
  accelerometer.y : Inport
  accelerometer.z : Inport  Port=2
  Discrete Derivative : simulink/Discrete/Discrete Derivative  gainval=1.0  ICPrevScaledInput=0  OutMin=[]  OutMax=[]  OutDataType=fixdt(1, 16)  OutScaling=2^-10  DoSatur=off
      settings: AttributesFormatString=initialCondition = %<ICPrevScaledInput>
  Discrete Filter: Bessel LPF : DiscreteFilter  Numerator=plant_mtr_encoder_filter_z_num  Denominator=plant_mtr_encoder_filter_z_den  SampleTime=mdl_T_sample
      settings: AttributesFormatString=|
      | Num: %<Numerator>
      | Den: %<Denominator>
  Trigonometric Function : Trigonometry  Operator=atan2
  " position.x" : Outport
  velocity.x : Outport  Port=2
  wires:
  accelerometer.y/1 -> Trigonometric Function/1
  accelerometer.z/1 -> Trigonometric Function/2
  Discrete Filter: Bessel LPF/1 -> velocity.x/1
  Trigonometric Function/1 -> Discrete Derivative/1, " position.x"/1
  Discrete Derivative/1 -> Discrete Filter: Bessel LPF/1

== system twr_2017a/Plant/Hardware/Calculations/Body Angular Position (phi)/X (Pitch)/Complementary Filter Gyroscope + Accelerometer (Incomplete) ==
  gyroscope.x : Inport
  accelerometer.y : Inport  Port=2
  accelerometer.z : Inport  Port=3
  Trigonometric Function : Trigonometry  Operator=atan2
  " position.x" : Outport
  velocity.x : Outport  Port=2
  wires:
  accelerometer.z/1 -> Trigonometric Function/2
  accelerometer.y/1 -> Trigonometric Function/1
  Trigonometric Function/1 -> ?
  gyroscope.x/1 -> ?

== system twr_2017a/Plant/Hardware/Calculations/Body Angular Position (phi)/X (Pitch)/Gyroscope ==
  gyroscope.x : Inport
  clock.timedEvent.plant.x_initialization : Inport  Port=2
  Discrete Filter: Bessel LPF : DiscreteFilter  Numerator=plant_gyro_filter_z_num  Denominator=plant_gyro_filter_z_den  SampleTime=mdl_T_sample
      settings: AttributesFormatString=|
      | Num: %<Numerator>
      | Den: %<Denominator>
  Discrete-Time Integrator : DiscreteIntegrator  ExternalReset=sampled level  SampleTime=-1  ICPrevOutput=DiscIntNeverNeededParam  ICPrevScaledInput=DiscIntNeverNeededParam
      settings: AttributesFormatString=initialCondition = %<InitialCondition>
  " position.x" : Outport
  velocity.x : Outport  Port=2
  wires:
  gyroscope.x/1 -> Discrete Filter: Bessel LPF/1
  Discrete-Time Integrator/1 -> " position.x"/1
  clock.timedEvent.plant.x_initialization/1 -> Discrete-Time Integrator/2
  Discrete Filter: Bessel LPF/1 -> Discrete-Time Integrator/1, velocity.x/1

== system twr_2017a/Plant/Hardware/Calculations/Body Angular Position (phi)/Y (Yaw)/Gyroscope ==
  gyroscope.y : Inport
  clock.timedEvent.plant.x_initialization : Inport  Port=2
  Discrete Filter: Bessel LPF : DiscreteFilter  Commented=through  Numerator=plant_gyro_encoder_filter_z_num  Denominator=plant_gyro_encoder_filter_z_den  SampleTime=mdl_T_sample
      settings: AttributesFormatString=|
      | Num: %<Numerator>
      | Den: %<Denominator>
  Discrete-Time Integrator : DiscreteIntegrator  ExternalReset=sampled level  SampleTime=-1  ICPrevOutput=DiscIntNeverNeededParam  ICPrevScaledInput=DiscIntNeverNeededParam
      settings: AttributesFormatString=initialCondition = %<InitialCondition>
  " position.y" : Outport
  velocity.y : Outport  Port=2
  wires:
  gyroscope.y/1 -> Discrete Filter: Bessel LPF/1
  Discrete-Time Integrator/1 -> " position.y"/1
  clock.timedEvent.plant.x_initialization/1 -> Discrete-Time Integrator/2
  Discrete Filter: Bessel LPF/1 -> Discrete-Time Integrator/1, velocity.y/1

== system twr_2017a/Plant/Hardware/Calculations/Body Angular Position (phi)/Y (Yaw)/Wheel Position ==
  wheel.angularPosition.global.left : Inport
  wheel.angularPosition.global.middle : Inport  Port=2
  Add : Sum  Inputs=-+
  Discrete Derivative : simulink/Discrete/Discrete Derivative  gainval=1.0  ICPrevScaledInput=0  OutMin=[]  OutMax=[]  OutDataType=fixdt(1, 16)  OutScaling=2^-10  DoSatur=off
      settings: AttributesFormatString=initialCondition = %<ICPrevScaledInput>
  Gain : Gain  Gain=plant_wheel_r / plant_body_l_w
      settings: AttributesFormatString=%<Gain>
  " position.y" : Outport
  " velocity.y" : Outport  Port=2
  wires:
  wheel.angularPosition.global.left/1 -> Add/1
  wheel.angularPosition.global.middle/1 -> Add/2
  Add/1 -> Gain/1
  Gain/1 -> Discrete Derivative/1, " position.y"/1
  Discrete Derivative/1 -> " velocity.y"/1

== system twr_2017a/Plant/Hardware/Calculations/Body Angular Position (phi)/Z (Roll)/Accelerometer ==
  accelerometer.x : Inport
  accelerometer.y : Inport  Port=2
  accelerometer.z : Inport  Port=3
  Add : Sum
  Derivative : Subsystem
  Gain : Gain  Gain=-1
  Math Function1 : Math  Operator=square  SignedPower=on  SaturateOnIntegerOverflow=on
  Math Function2 : Math  Operator=square  SignedPower=on  SaturateOnIntegerOverflow=on
  Sqrt : Sqrt  SaturateOnIntegerOverflow=on
  Trigonometric Function : Trigonometry  Operator=atan2
  position.z : Outport
  velocity.z : Outport  Port=2
  wires:
  accelerometer.y/1 -> Math Function1/1
  Math Function1/1 -> Add/1
  Sqrt/1 -> Trigonometric Function/2
  accelerometer.z/1 -> Math Function2/1
  accelerometer.x/1 -> Gain/1
  Gain/1 -> Trigonometric Function/1
  Math Function2/1 -> Add/2
  Trigonometric Function/1 -> Derivative/1(x), position.z/1
  Add/1 -> Sqrt/1
  Derivative/1(x.dot) -> velocity.z/1

== system twr_2017a/Plant/Hardware/Calculations/Body Angular Position (phi)/Z (Roll)/Complementary Filter Gyroscope + Accelerometer (Incomplete) ==
  gyroscope.z : Inport
  accelerometer.x : Inport  Port=2
  accelerometer.y : Inport  Port=3
  accelerometer.z : Inport  Port=4
  Add : Sum
  Gain : Gain  Gain=-1
  Math Function1 : Math  Operator=square  SignedPower=on  SaturateOnIntegerOverflow=on
  Math Function2 : Math  Operator=square  SignedPower=on  SaturateOnIntegerOverflow=on
  Sqrt : Sqrt  SaturateOnIntegerOverflow=on
  Trigonometric Function : Trigonometry  Operator=atan2
  position.z : Outport
  velocity.z : Outport  Port=2
  wires:
  gyroscope.z/1 -> ?
  accelerometer.y/1 -> Math Function1/1
  accelerometer.x/1 -> Gain/1
  Gain/1 -> Trigonometric Function/1
  Math Function1/1 -> Add/1
  Sqrt/1 -> Trigonometric Function/2
  accelerometer.z/1 -> Math Function2/1
  Math Function2/1 -> Add/2
  Add/1 -> Sqrt/1
  Trigonometric Function/1 -> ?

== system twr_2017a/Plant/Hardware/Calculations/Body Angular Position (phi)/Z (Roll)/Gyroscope ==
  gyroscope.z : Inport
  clock.timedEvent.plant.x_initialization : Inport  Port=2
  Discrete Filter: Bessel LPF : DiscreteFilter  Numerator=plant_gyro_filter_z_num  Denominator=plant_gyro_filter_z_den  SampleTime=mdl_T_sample
      settings: AttributesFormatString=|
      | Num: %<Numerator>
      | Den: %<Denominator>
  Discrete-Time Integrator : DiscreteIntegrator  ExternalReset=sampled level  SampleTime=-1  ICPrevOutput=DiscIntNeverNeededParam  ICPrevScaledInput=DiscIntNeverNeededParam
      settings: AttributesFormatString=initialCondition = %<InitialCondition>
  " position.z" : Outport
  velocity.z : Outport  Port=2
  wires:
  gyroscope.z/1 -> Discrete Filter: Bessel LPF/1
  Discrete-Time Integrator/1 -> " position.z"/1
  clock.timedEvent.plant.x_initialization/1 -> Discrete-Time Integrator/2
  Discrete Filter: Bessel LPF/1 -> Discrete-Time Integrator/1, velocity.z/1

== system twr_2017a/Plant/Hardware/Calculations/Linear Position (p)/Wheel/Center ==
  wheel.angularVelocity.global : Inport
  body.angularPosition.y (yaw) : Inport  Port=2
  Add1 : Sum
  Bus Creator : BusCreator  Inputs=2
  Bus Creator1 : BusCreator  Inputs=2
  Bus Creator2 : BusCreator  Inputs=2
  Constant : Constant  Value=0  SampleTime=mdl_T_sample
  Constant1 : Constant  Value=plant_wheel_r / 2  SampleTime=mdl_T_sample
      settings: AttributesFormatString=%<Value>
  Discrete-Time Integrator [x] : DiscreteIntegrator  SampleTime=-1  ICPrevOutput=DiscIntNeverNeededParam  ICPrevScaledInput=DiscIntNeverNeededParam
      settings: AttributesFormatString=initialCondition = %<InitialCondition>
  Discrete-Time Integrator [y] : DiscreteIntegrator  SampleTime=-1  ICPrevOutput=DiscIntNeverNeededParam  ICPrevScaledInput=DiscIntNeverNeededParam
      settings: AttributesFormatString=initialCondition = %<InitialCondition>
  Discrete-Time Integrator [z] : DiscreteIntegrator  SampleTime=-1  ICPrevOutput=DiscIntNeverNeededParam  ICPrevScaledInput=DiscIntNeverNeededParam
      settings: AttributesFormatString=initialCondition = %<InitialCondition>
  Gain3 : Gain  Gain=plant_wheel_r
      settings: AttributesFormatString=%<Gain>
  Gain4 : Gain  Gain=plant_wheel_r
      settings: AttributesFormatString=%<Gain>
  Product : Product
  Product1 : Product
  Trigonometric Function : Trigonometry  Operator=cos
  Trigonometric Function1 : Trigonometry
  x : Outport
  y : Outport  Port=2
  z : Outport  Port=3
  wires:
  Bus Creator2/1 -> z/1
  Bus Creator/1 -> x/1
  Bus Creator1/1 -> y/1
  Product/1 -> Discrete-Time Integrator [x]/1, Bus Creator/2  "velocity [m/s]"
  Product1/1 -> Discrete-Time Integrator [y]/1, Bus Creator1/2  "velocity [m/s]"
  Constant/1 -> Discrete-Time Integrator [z]/1, Bus Creator2/2  "velocity [m/s]"
  Discrete-Time Integrator [x]/1 -> Bus Creator/1  "position [m]"
  Discrete-Time Integrator [y]/1 -> Bus Creator1/1  "position [m]"
  Add1/1 -> Bus Creator2/1  "position [m]"
  wheel.angularVelocity.global/1 -> [theta_dot]
  Gain3/1 -> Product/1
  Trigonometric Function/1 -> Product/2
  body.angularPosition.y (yaw)/1 -> [yaw]
  Trigonometric Function1/1 -> Product1/2
  Gain4/1 -> Product1/1
  [yaw] -> Trigonometric Function/1
  [theta_dot] -> Gain3/1
  [theta_dot] -> Gain4/1
  [yaw] -> Trigonometric Function1/1
  Discrete-Time Integrator [z]/1 -> Add1/2
  Constant1/1 -> Add1/1

== system twr_2017a/Plant/Hardware/Calculations/Linear Position (p)/Wheel/Left-Connected ==
  p.center.x : Inport
  p.center.y : Inport  Port=2
  p.center.z : Inport  Port=3
  body.angularPosition.y (yaw) : Inport  Port=4
  Add1 : Sum
  Add2 : Sum
  Bus Creator : BusCreator  Inputs=2
  Bus Creator1 : BusCreator  Inputs=2
  Bus Creator2 : BusCreator  Inputs=2
  Discrete Derivative [Average] : simulink/Discrete/Discrete Derivative  gainval=1.0  ICPrevScaledInput=0  OutMin=[]  OutMax=[]  OutDataType=fixdt(1, 16)  OutScaling=2^-10  DoSatur=off
      settings: AttributesFormatString=initialCondition = %<ICPrevScaledInput>
  Discrete Derivative [Left-Connected] : simulink/Discrete/Discrete Derivative  gainval=1.0  ICPrevScaledInput=0  OutMin=[]  OutMax=[]  OutDataType=fixdt(1, 16)  OutScaling=2^-10  DoSatur=off
      settings: AttributesFormatString=initialCondition = %<ICPrevScaledInput>
  Discrete Derivative [Middle-Connected] : simulink/Discrete/Discrete Derivative  gainval=1.0  ICPrevScaledInput=0  OutMin=[]  OutMax=[]  OutDataType=fixdt(1, 16)  OutScaling=2^-10  DoSatur=off
      settings: AttributesFormatString=initialCondition = %<ICPrevScaledInput>
  Gain3 : Gain  Gain=- plant_body_l_w / 2
      settings: AttributesFormatString=%<Gain>
  Gain4 : Gain  Gain=+ plant_body_l_w / 2
      settings: AttributesFormatString=%<Gain>
  Trigonometric Function : Trigonometry
  Trigonometric Function1 : Trigonometry  Operator=cos
  x : Outport
  y : Outport  Port=2
  z : Outport  Port=3
  wires:
  Gain4/1 -> Add2/2
  Gain3/1 -> Add1/2
  [yaw] -> Trigonometric Function1/1
  body.angularPosition.y (yaw)/1 -> [yaw]
  p.center.y/1 -> Add2/1
  Trigonometric Function1/1 -> Gain4/1
  p.center.x/1 -> Add1/1
  Trigonometric Function/1 -> Gain3/1
  [yaw] -> Trigonometric Function/1
  Add1/1 -> Discrete Derivative [Left-Connected]/1, Bus Creator/1  "position [m]"
  Add2/1 -> Bus Creator1/1, Discrete Derivative [Middle-Connected]/1  "position [m]"
  Bus Creator2/1 -> z/1
  p.center.z/1 -> Discrete Derivative [Average]/1, Bus Creator2/1  "position [m]"
  Bus Creator/1 -> x/1
  Bus Creator1/1 -> y/1
  Discrete Derivative [Left-Connected]/1 -> Bus Creator/2  "velocity [m/s]"
  Discrete Derivative [Middle-Connected]/1 -> Bus Creator1/2  "velocity [m/s]"
  Discrete Derivative [Average]/1 -> Bus Creator2/2  "velocity [m/s]"
